simulink model "ODE_Hand_Model_v08_IPC_v03"  (Simulink 7.5)
settings: Solver=FixedStepDiscrete  StartTime=0.0  StopTime=inf  FixedStep=0.0315/(4*12)  RelTol=1e-3
values from neighbouring files (symbols this model uses):
  f_step = 0.7    [Set_Parameters.m]
  force_step = 20    [Set_Parameters.m]
  K_Conn = eye(4)*k_conn    [Set_Parameters.m]
  K_D = 30    [Set_Parameters.m]
  K_Or = eye(3)*k_Or    [Set_Parameters.m]
  K_Ot = eye(3)*k_Ot    [Set_Parameters.m]
  K_P = 350    [Set_Parameters.m]
  ksi = 0.9    [Set_Parameters.m]
  Kx = diag([diag(K_Ot)' diag(K_Or)' diag(K_Conn)'])    [Set_Parameters.m]
  l_des = [l1_des; l2_des; l3_des; l4_des]    [Set_Parameters.m]
  Mo = diag([sphere_mass*ones(1,3) (2/5)*sphere_mass*sphere_radius^2*ones(1,3)])    [Set_Parameters.m]
  qd_initial_touch = [0 0.3655   -0.5897   -0.5897     0       -0.3333   +0.5942   +0.5942         0       -0.298   --0.5226   --0.5226           0       -0.3333   +0.5942   +0.5942]    [Set_Parameters.m]
  R_O_Desired = R_O(x_i_v02(qd_initial_touch))    [Set_Parameters.m]
  t_f_start = 2.5    [Set_Parameters.m]
  torque_step = 60    [Set_Parameters.m]
  x_O_desired = (1/4)*sum(x_i_v02(qd_initial_touch))    [Set_Parameters.m]
undefined symbols (not defined in the file or in its folder): sigbuilder_block
libraries: dspmtrx3 x33, simulink x2, dspinverses x1
(part 6 of 6)

== matlab function Control/IPC/J/J_Or1/Embedded MATLAB Function2 ==
  data: xi input double size=[4 3]; J_r3 output double
%#eml
function J_r3 = partial_r3_to_x(xi)


x1 = xi(1,:)';
x2 = xi(2,:)';
x3 = xi(3,:)';
x4 = xi(4,:)';

r1=(( x1-x3 )/norm( x1-x3 ) + ...
    ( x2-x4 )/norm( x2-x4 ));


r1_unit=(r1/norm(r1));

r3 = skew( x1-x3 ) * ( x2-x4 );
r3_unit=r3/norm(r3);

r2_unit = skew(r3_unit)*r1_unit;

% RO=[r1_unit r2_unit r3_unit];


% partial_r3__term1 = (((norm(r3)^2)*eye(3)-(r3)*(r3)') / (norm((r3))^3));
partial_r3__term1 = (-skew(r3)^2)/(norm(r3)^3);

partial_r3__term2_x1x3 = skew(x2-x4)';
partial_r3__term2_x2x4 =  skew(x1-x3); 

partial_r3__term3_x1x2 =  eye(3);
partial_r3__term3_x3x4 = -eye(3);

J_r3_x1 = partial_r3__term1*partial_r3__term2_x1x3*partial_r3__term3_x1x2;

J_r3_x2 = partial_r3__term1*partial_r3__term2_x2x4*partial_r3__term3_x1x2;
       
J_r3_x3 = partial_r3__term1*partial_r3__term2_x1x3*partial_r3__term3_x3x4;
                    
J_r3_x4 = partial_r3__term1*partial_r3__term2_x2x4*partial_r3__term3_x3x4;


J_r3 = [J_r3_x1,J_r3_x2,J_r3_x3,J_r3_x4];

== matlab function Control/IPC/J/J_Or1/Embedded MATLAB Function3 ==
  data: xi input double size=[4 3]; J_r1 output double
%#eml
function J_r1 = partial_r1_to_x(xi)


x1 = xi(1,:)';
x2 = xi(2,:)';
x3 = xi(3,:)';
x4 = xi(4,:)';

r1=(( x1-x3 )/norm( x1-x3 ) + ( x2-x4 )/norm( x2-x4 ));

% r1=(( x1-x3 )/norm( x1-x3 ) + ( x2-x4 ))


r1_unit=(r1/norm(r1));

r3= skew( x1-x3 ) * ( x2-x4 );
r3_unit=r3/norm(r3);

r2_unit = skew(r3_unit)*r1_unit;

% RO=[r1_unit r2_unit r3_unit];


% partial_r1__term1 = (((norm(r1)^2)*eye(3)-(r1)*(r1)') / (norm((r1))^3));
partial_r1__term1 = (-skew(r1)^2)/(norm(r1)^3);

partial_r1__term2_x1x3 = (((norm((x1-x3))^2)*eye(3)-(x1-x3)*(x1-x3)') / (norm((x1-x3))^3));
partial_r1__term2_x2x4 = (((norm((x2-x4))^2)*eye(3)-(x2-x4)*(x2-x4)') / (norm((x2-x4))^3));


partial_r1__term3_x1x2 = eye(3);
partial_r1__term3_x3x4 = -eye(3);



J_r1_x1 = partial_r1__term1*partial_r1__term2_x1x3*partial_r1__term3_x1x2;

J_r2 = skew(r3_unit)*J_r1_x1';

J_r1_x2 = partial_r1__term1*partial_r1__term2_x2x4*partial_r1__term3_x1x2;
       
J_r1_x3 = partial_r1__term1*partial_r1__term2_x1x3*partial_r1__term3_x3x4;
       
J_r1_x4 = partial_r1__term1*partial_r1__term2_x2x4*partial_r1__term3_x3x4;


% J_r1_x1 = [partial_r1__term1.*partial_r1__term2_x1x3.*partial_r1__term3_x1x2(:,1), ...
%            partial_r1__term1.*partial_r1__term2_x1x3.*partial_r1__term3_x1x2(:,2), ...
%            partial_r1__term1.*partial_r1__term2_x1x3.*partial_r1__term3_x1x2(:,3)];
% 
% J_r1_x2 = [partial_r1__term1.*partial_r1__term2_x2x4.*partial_r1__term3_x1x2(:,1), ...
%            partial_r1__term1.*partial_r1__term2_x2x4.*partial_r1__term3_x1x2(:,2), ...
%            partial_r1__term1.*partial_r1__term2_x2x4.*partial_r1__term3_x1x2(:,3)];
%        
% J_r1_x3 = [partial_r1__term1.*partial_r1__term2_x1x3.*partial_r1__term3_x3x4(:,1), ...
%            partial_r1__term1.*partial_r1__term2_x1x3.*partial_r1__term3_x3x4(:,2), ...
%            partial_r1__term1.*partial_r1__term2_x1x3.*partial_r1__term3_x3x4(:,3)];
%        
% J_r1_x4 = [partial_r1__term1.*partial_r1__term2_x2x4.*partial_r1__term3_x3x4(:,1), ...
%            partial_r1__term1.*partial_r1__term2_x2x4.*partial_r1__term3_x3x4(:,2), ...
%            partial_r1__term1.*partial_r1__term2_x2x4.*partial_r1__term3_x3x4(:,3)];

J_r1 = [J_r1_x1,J_r1_x2,J_r1_x3,J_r1_x4];

== matlab function Control/IPC/Object Level Damping(theta)/Embedded MATLAB Function ==
  data: q input double; M output double
%#eml
function M=Inertia_Dynamic_Terms(q)

M1=zeros(16);

L1 = 0.10;
L2 = 1.10;
L3 = 0.60;
L4 = 0.55;

capsule1Inertia = 0.1675;
capsule2Inertia = 0.0837;
capsule3Inertia = 0.0834;

caspule1mass = 2.00;
caspule2mass = 1.00;
caspule3mass = 1.00;

for i=1:4:16,
q1 = q(i);
q2 = q(i+1);
q3 = q(i+2);
q4 = q(i+3);
    
    
M1(i:i+3,i:i+3)=[capsule1Inertia .* cos(q2) .^ 2 + capsule2Inertia .* cos(q2 + q3) ...
   .^ 2 + capsule3Inertia .* cos(q2 + q3 + q4) .^ 2 + caspule1mass  ...
  .* ((1 / 4) .* L2 .^ 2 .* cos(q1) .^ 2 .* cos(q2) .^ 2 + (1 / 4)  ...
  .* L2 .^ 2 .* cos(q2) .^ 2 .* sin(q1) .^ 2) + caspule2mass .* ((( ...
  -1 / 2) .* L3 .* cos(q1) .* cos(q2 + q3) + cos(q1) .* (L2 .* cos( ...
  q2) + L3 .* cos(q2 + q3))) .^ 2 + ((1 / 2) .* L3 .* cos(q2 + q3)  ...
  .* sin(q1) + (-1) .* (L2 .* cos(q2) + L3 .* cos(q2 + q3)) .* sin( ...
  q1)) .^ 2) + caspule3mass .* (((-1 / 2) .* L4 .* cos(q1) .* cos( ...
  q2 + q3 + q4) + cos(q1) .* (L2 .* cos(q2) + L3 .* cos(q2 + q3) +  ...
  L4 .* cos(q2 + q3 + q4))) .^ 2 + ((1 / 2) .* L4 .* cos(q2 + q3 +  ...
  q4) .* sin(q1) + (-1) .* (L2 .* cos(q2) + L3 .* cos(q2 + q3) + L4  ...
  .* cos(q2 + q3 + q4)) .* sin(q1)) .^ 2) + capsule1Inertia .* sin( ...
  q2) .^ 2 + capsule2Inertia .* sin(q2 + q3) .^ 2 + capsule3Inertia  ...
  .* sin(q2 + q3 + q4) .^ 2,caspule2mass .* ((-1) .* ((-1 / 2) .*  ...
  L3 .* cos(q1) .* cos(q2 + q3) + cos(q1) .* (L2 .* cos(q2) + L3 .*  ...
  cos(q2 + q3))) .* sin(q1) .* (L2 .* sin(q2) + (1 / 2) .* L3 .*  ...
  sin(q2 + q3)) + (-1) .* cos(q1) .* ((1 / 2) .* L3 .* cos(q2 + q3)  ...
  .* sin(q1) + (-1) .* (L2 .* cos(q2) + L3 .* cos(q2 + q3)) .* sin( ...
  q1)) .* (L2 .* sin(q2) + (1 / 2) .* L3 .* sin(q2 + q3))) +  ...
  caspule3mass .* ((-1) .* ((-1 / 2) .* L4 .* cos(q1) .* cos(q2 +  ...
  q3 + q4) + cos(q1) .* (L2 .* cos(q2) + L3 .* cos(q2 + q3) + L4 .*  ...
  cos(q2 + q3 + q4))) .* sin(q1) .* (L2 .* sin(q2) + L3 .* sin(q2 +  ...
  q3) + (1 / 2) .* L4 .* sin(q2 + q3 + q4)) + (-1) .* cos(q1) .* (( ...
  1 / 2) .* L4 .* cos(q2 + q3 + q4) .* sin(q1) + (-1) .* (L2 .* cos( ...
  q2) + L3 .* cos(q2 + q3) + L4 .* cos(q2 + q3 + q4)) .* sin(q1)) .* ...
   (L2 .* sin(q2) + L3 .* sin(q2 + q3) + (1 / 2) .* L4 .* sin(q2 +  ...
  q3 + q4))),caspule2mass .* ((-1 / 2) .* L3 .* ((-1 / 2) .* L3 .*  ...
  cos(q1) .* cos(q2 + q3) + cos(q1) .* (L2 .* cos(q2) + L3 .* cos( ...
  q2 + q3))) .* sin(q1) .* sin(q2 + q3) + (-1 / 2) .* L3 .* cos(q1)  ...
  .* ((1 / 2) .* L3 .* cos(q2 + q3) .* sin(q1) + (-1) .* (L2 .* cos( ...
  q2) + L3 .* cos(q2 + q3)) .* sin(q1)) .* sin(q2 + q3)) +  ...
  caspule3mass .* ((-1) .* ((-1 / 2) .* L4 .* cos(q1) .* cos(q2 +  ...
  q3 + q4) + cos(q1) .* (L2 .* cos(q2) + L3 .* cos(q2 + q3) + L4 .*  ...
  cos(q2 + q3 + q4))) .* sin(q1) .* (L3 .* sin(q2 + q3) + (1 / 2) .* ...
   L4 .* sin(q2 + q3 + q4)) + (-1) .* cos(q1) .* ((1 / 2) .* L4 .*  ...
  cos(q2 + q3 + q4) .* sin(q1) + (-1) .* (L2 .* cos(q2) + L3 .* cos( ...
  q2 + q3) + L4 .* cos(q2 + q3 + q4)) .* sin(q1)) .* (L3 .* sin(q2 + ...
   q3) + (1 / 2) .* L4 .* sin(q2 + q3 + q4))),caspule3mass .* ((-1  ...
  / 2) .* L4 .* ((-1 / 2) .* L4 .* cos(q1) .* cos(q2 + q3 + q4) +  ...
  cos(q1) .* (L2 .* cos(q2) + L3 .* cos(q2 + q3) + L4 .* cos(q2 +  ...
  q3 + q4))) .* sin(q1) .* sin(q2 + q3 + q4) + (-1 / 2) .* L4 .*  ...
  cos(q1) .* ((1 / 2) .* L4 .* cos(q2 + q3 + q4) .* sin(q1) + (-1)  ...
  .* (L2 .* cos(q2) + L3 .* cos(q2 + q3) + L4 .* cos(q2 + q3 + q4))  ...
  .* sin(q1)) .* sin(q2 + q3 + q4));caspule2mass .* ((-1) .* ((-1 /  ...
  2) .* L3 .* cos(q1) .* cos(q2 + q3) + cos(q1) .* (L2 .* cos(q2) +  ...
  L3 .* cos(q2 + q3))) .* sin(q1) .* (L2 .* sin(q2) + (1 / 2) .* L3  ...
  .* sin(q2 + q3)) + (-1) .* cos(q1) .* ((1 / 2) .* L3 .* cos(q2 +  ...
  q3) .* sin(q1) + (-1) .* (L2 .* cos(q2) + L3 .* cos(q2 + q3)) .*  ...
  sin(q1)) .* (L2 .* sin(q2) + (1 / 2) .* L3 .* sin(q2 + q3))) +  ...
  caspule3mass .* ((-1) .* ((-1 / 2) .* L4 .* cos(q1) .* cos(q2 +  ...
  q3 + q4) + cos(q1) .* (L2 .* cos(q2) + L3 .* cos(q2 + q3) + L4 .*  ...
  cos(q2 + q3 + q4))) .* sin(q1) .* (L2 .* sin(q2) + L3 .* sin(q2 +  ...
  q3) + (1 / 2) .* L4 .* sin(q2 + q3 + q4)) + (-1) .* cos(q1) .* (( ...
  1 / 2) .* L4 .* cos(q2 + q3 + q4) .* sin(q1) + (-1) .* (L2 .* cos( ...
  q2) + L3 .* cos(q2 + q3) + L4 .* cos(q2 + q3 + q4)) .* sin(q1)) .* ...
   (L2 .* sin(q2) + L3 .* sin(q2 + q3) + (1 / 2) .* L4 .* sin(q2 +  ...
  q3 + q4))),capsule1Inertia .* cos(q1) .^ 2 .* (cos(q1) .^ 2 + sin( ...
  q1) .^ 2) + capsule2Inertia .* cos(q1) .^ 2 .* (cos(q1) .^ 2 +  ...
  sin(q1) .^ 2) + capsule3Inertia .* cos(q1) .^ 2 .* (cos(q1) .^ 2 + ...
   sin(q1) .^ 2) + capsule1Inertia .* sin(q1) .^ 2 .* (cos(q1) .^ 2  ...
  + sin(q1) .^ 2) + capsule2Inertia .* sin(q1) .^ 2 .* (cos(q1) .^  ...
  2 + sin(q1) .^ 2) + capsule3Inertia .* sin(q1) .^ 2 .* (cos(q1)  ...
  .^ 2 + sin(q1) .^ 2) + caspule1mass .* (((1 / 2) .* L2 .* cos(q1)  ...
  .^ 2 .* cos(q2) + (1 / 2) .* L2 .* cos(q2) .* sin(q1) .^ 2) .^ 2 + ...
   (1 / 4) .* L2 .^ 2 .* cos(q1) .^ 2 .* sin(q2) .^ 2 + (1 / 4) .*  ...
  L2 .^ 2 .* sin(q1) .^ 2 .* sin(q2) .^ 2) + caspule2mass .* ((cos( ...
  q1) .* ((-1 / 2) .* L3 .* cos(q1) .* cos(q2 + q3) + cos(q1) .* ( ...
  L2 .* cos(q2) + L3 .* cos(q2 + q3))) + sin(q1) .* ((-1 / 2) .* L3  ...
  .* cos(q2 + q3) .* sin(q1) + (L2 .* cos(q2) + L3 .* cos(q2 + q3))  ...
  .* sin(q1))) .^ 2 + cos(q1) .^ 2 .* (L2 .* sin(q2) + (1 / 2) .*  ...
  L3 .* sin(q2 + q3)) .^ 2 + sin(q1) .^ 2 .* (L2 .* sin(q2) + (1 /  ...
  2) .* L3 .* sin(q2 + q3)) .^ 2) + caspule3mass .* ((cos(q1) .* (( ...
  -1 / 2) .* L4 .* cos(q1) .* cos(q2 + q3 + q4) + cos(q1) .* (L2 .*  ...
  cos(q2) + L3 .* cos(q2 + q3) + L4 .* cos(q2 + q3 + q4))) + sin(q1) ...
   .* ((-1 / 2) .* L4 .* cos(q2 + q3 + q4) .* sin(q1) + (L2 .* cos( ...
  q2) + L3 .* cos(q2 + q3) + L4 .* cos(q2 + q3 + q4)) .* sin(q1)))  ...
  .^ 2 + cos(q1) .^ 2 .* (L2 .* sin(q2) + L3 .* sin(q2 + q3) + (1 /  ...
  2) .* L4 .* sin(q2 + q3 + q4)) .^ 2 + sin(q1) .^ 2 .* (L2 .* sin( ...
  q2) + L3 .* sin(q2 + q3) + (1 / 2) .* L4 .* sin(q2 + q3 + q4)) .^  ...
  2),capsule2Inertia .* cos(q1) .^ 2 .* (cos(q1) .^ 2 + sin(q1) .^  ...
  2) + capsule3Inertia .* cos(q1) .^ 2 .* (cos(q1) .^ 2 + sin(q1)  ...
  .^ 2) + capsule2Inertia .* sin(q1) .^ 2 .* (cos(q1) .^ 2 + sin(q1) ...
   .^ 2) + capsule3Inertia .* sin(q1) .^ 2 .* (cos(q1) .^ 2 + sin( ...
  q1) .^ 2) + caspule2mass .* ((cos(q1) .* ((-1 / 2) .* L3 .* cos( ...
  q1) .* cos(q2 + q3) + cos(q1) .* (L2 .* cos(q2) + L3 .* cos(q2 +  ...
  q3))) + sin(q1) .* ((-1 / 2) .* L3 .* cos(q2 + q3) .* sin(q1) + ( ...
  L2 .* cos(q2) + L3 .* cos(q2 + q3)) .* sin(q1))) .* (cos(q1) .* (( ...
  -1) .* L2 .* cos(q1) .* cos(q2) + (-1 / 2) .* L3 .* cos(q1) .*  ...
  cos(q2 + q3) + cos(q1) .* (L2 .* cos(q2) + L3 .* cos(q2 + q3))) +  ...
  sin(q1) .* ((-1) .* L2 .* cos(q2) .* sin(q1) + (-1 / 2) .* L3 .*  ...
  cos(q2 + q3) .* sin(q1) + (L2 .* cos(q2) + L3 .* cos(q2 + q3)) .*  ...
  sin(q1))) + (1 / 2) .* L3 .* cos(q1) .^ 2 .* sin(q2 + q3) .* (L2  ...
  .* sin(q2) + (1 / 2) .* L3 .* sin(q2 + q3)) + (1 / 2) .* L3 .*  ...
  sin(q1) .^ 2 .* sin(q2 + q3) .* (L2 .* sin(q2) + (1 / 2) .* L3 .*  ...
  sin(q2 + q3))) + caspule3mass .* ((cos(q1) .* ((-1 / 2) .* L4 .*  ...
  cos(q1) .* cos(q2 + q3 + q4) + cos(q1) .* (L2 .* cos(q2) + L3 .*  ...
  cos(q2 + q3) + L4 .* cos(q2 + q3 + q4))) + sin(q1) .* ((-1 / 2) .* ...
   L4 .* cos(q2 + q3 + q4) .* sin(q1) + (L2 .* cos(q2) + L3 .* cos( ...
  q2 + q3) + L4 .* cos(q2 + q3 + q4)) .* sin(q1))) .* (cos(q1) .* (( ...
  -1) .* L2 .* cos(q1) .* cos(q2) + (-1 / 2) .* L4 .* cos(q1) .*  ...
  cos(q2 + q3 + q4) + cos(q1) .* (L2 .* cos(q2) + L3 .* cos(q2 + q3) ...
   + L4 .* cos(q2 + q3 + q4))) + sin(q1) .* ((-1) .* L2 .* cos(q2)  ...
  .* sin(q1) + (-1 / 2) .* L4 .* cos(q2 + q3 + q4) .* sin(q1) + (L2  ...
  .* cos(q2) + L3 .* cos(q2 + q3) + L4 .* cos(q2 + q3 + q4)) .* sin( ...
  q1))) + cos(q1) .^ 2 .* (L3 .* sin(q2 + q3) + (1 / 2) .* L4 .*  ...
  sin(q2 + q3 + q4)) .* (L2 .* sin(q2) + L3 .* sin(q2 + q3) + (1 /  ...
  2) .* L4 .* sin(q2 + q3 + q4)) + sin(q1) .^ 2 .* (L3 .* sin(q2 +  ...
  q3) + (1 / 2) .* L4 .* sin(q2 + q3 + q4)) .* (L2 .* sin(q2) + L3  ...
  .* sin(q2 + q3) + (1 / 2) .* L4 .* sin(q2 + q3 + q4))), ...
  capsule3Inertia .* cos(q1) .^ 2 .* (cos(q1) .^ 2 + sin(q1) .^ 2) + ...
   capsule3Inertia .* sin(q1) .^ 2 .* (cos(q1) .^ 2 + sin(q1) .^ 2)  ...
  + caspule3mass .* ((cos(q1) .* ((-1 / 2) .* L4 .* cos(q1) .* cos( ...
  q2 + q3 + q4) + cos(q1) .* (L2 .* cos(q2) + L3 .* cos(q2 + q3) +  ...
  L4 .* cos(q2 + q3 + q4))) + sin(q1) .* ((-1 / 2) .* L4 .* cos(q2 + ...
   q3 + q4) .* sin(q1) + (L2 .* cos(q2) + L3 .* cos(q2 + q3) + L4 .* ...
   cos(q2 + q3 + q4)) .* sin(q1))) .* (cos(q1) .* ((-1) .* cos(q1)  ...
  .* (L2 .* cos(q2) + L3 .* cos(q2 + q3)) + (-1 / 2) .* L4 .* cos( ...
  q1) .* cos(q2 + q3 + q4) + cos(q1) .* (L2 .* cos(q2) + L3 .* cos( ...
  q2 + q3) + L4 .* cos(q2 + q3 + q4))) + sin(q1) .* ((-1) .* (L2 .*  ...
  cos(q2) + L3 .* cos(q2 + q3)) .* sin(q1) + (-1 / 2) .* L4 .* cos( ...
  q2 + q3 + q4) .* sin(q1) + (L2 .* cos(q2) + L3 .* cos(q2 + q3) +  ...
  L4 .* cos(q2 + q3 + q4)) .* sin(q1))) + (1 / 2) .* L4 .* cos(q1)  ...
  .^ 2 .* sin(q2 + q3 + q4) .* (L2 .* sin(q2) + L3 .* sin(q2 + q3) + ...
   (1 / 2) .* L4 .* sin(q2 + q3 + q4)) + (1 / 2) .* L4 .* sin(q1)  ...
  .^ 2 .* sin(q2 + q3 + q4) .* (L2 .* sin(q2) + L3 .* sin(q2 + q3) + ...
   (1 / 2) .* L4 .* sin(q2 + q3 + q4)));caspule2mass .* ((-1 / 2) .* ...
   L3 .* ((-1 / 2) .* L3 .* cos(q1) .* cos(q2 + q3) + cos(q1) .* ( ...
  L2 .* cos(q2) + L3 .* cos(q2 + q3))) .* sin(q1) .* sin(q2 + q3) +  ...
  (-1 / 2) .* L3 .* cos(q1) .* ((1 / 2) .* L3 .* cos(q2 + q3) .*  ...
  sin(q1) + (-1) .* (L2 .* cos(q2) + L3 .* cos(q2 + q3)) .* sin(q1)) ...
   .* sin(q2 + q3)) + caspule3mass .* ((-1) .* ((-1 / 2) .* L4 .*  ...
  cos(q1) .* cos(q2 + q3 + q4) + cos(q1) .* (L2 .* cos(q2) + L3 .*  ...
  cos(q2 + q3) + L4 .* cos(q2 + q3 + q4))) .* sin(q1) .* (L3 .* sin( ...
  q2 + q3) + (1 / 2) .* L4 .* sin(q2 + q3 + q4)) + (-1) .* cos(q1)  ...
  .* ((1 / 2) .* L4 .* cos(q2 + q3 + q4) .* sin(q1) + (-1) .* (L2 .* ...
   cos(q2) + L3 .* cos(q2 + q3) + L4 .* cos(q2 + q3 + q4)) .* sin( ...
  q1)) .* (L3 .* sin(q2 + q3) + (1 / 2) .* L4 .* sin(q2 + q3 + q4))) ...
  ,capsule2Inertia .* cos(q1) .^ 2 .* (cos(q1) .^ 2 + sin(q1) .^ 2)  ...
  + capsule3Inertia .* cos(q1) .^ 2 .* (cos(q1) .^ 2 + sin(q1) .^ 2) ...
   + capsule2Inertia .* sin(q1) .^ 2 .* (cos(q1) .^ 2 + sin(q1) .^  ...
  2) + capsule3Inertia .* sin(q1) .^ 2 .* (cos(q1) .^ 2 + sin(q1)  ...
  .^ 2) + caspule2mass .* ((cos(q1) .* ((-1 / 2) .* L3 .* cos(q1) .* ...
   cos(q2 + q3) + cos(q1) .* (L2 .* cos(q2) + L3 .* cos(q2 + q3))) + ...
   sin(q1) .* ((-1 / 2) .* L3 .* cos(q2 + q3) .* sin(q1) + (L2 .*  ...
  cos(q2) + L3 .* cos(q2 + q3)) .* sin(q1))) .* (cos(q1) .* ((-1) .* ...
   L2 .* cos(q1) .* cos(q2) + (-1 / 2) .* L3 .* cos(q1) .* cos(q2 +  ...
  q3) + cos(q1) .* (L2 .* cos(q2) + L3 .* cos(q2 + q3))) + sin(q1)  ...
  .* ((-1) .* L2 .* cos(q2) .* sin(q1) + (-1 / 2) .* L3 .* cos(q2 +  ...
  q3) .* sin(q1) + (L2 .* cos(q2) + L3 .* cos(q2 + q3)) .* sin(q1))) ...
   + (1 / 2) .* L3 .* cos(q1) .^ 2 .* sin(q2 + q3) .* (L2 .* sin(q2) ...
   + (1 / 2) .* L3 .* sin(q2 + q3)) + (1 / 2) .* L3 .* sin(q1) .^ 2  ...
  .* sin(q2 + q3) .* (L2 .* sin(q2) + (1 / 2) .* L3 .* sin(q2 + q3)) ...
  ) + caspule3mass .* ((cos(q1) .* ((-1 / 2) .* L4 .* cos(q1) .*  ...
  cos(q2 + q3 + q4) + cos(q1) .* (L2 .* cos(q2) + L3 .* cos(q2 + q3) ...
   + L4 .* cos(q2 + q3 + q4))) + sin(q1) .* ((-1 / 2) .* L4 .* cos( ...
  q2 + q3 + q4) .* sin(q1) + (L2 .* cos(q2) + L3 .* cos(q2 + q3) +  ...
  L4 .* cos(q2 + q3 + q4)) .* sin(q1))) .* (cos(q1) .* ((-1) .* L2  ...
  .* cos(q1) .* cos(q2) + (-1 / 2) .* L4 .* cos(q1) .* cos(q2 + q3 + ...
   q4) + cos(q1) .* (L2 .* cos(q2) + L3 .* cos(q2 + q3) + L4 .* cos( ...
  q2 + q3 + q4))) + sin(q1) .* ((-1) .* L2 .* cos(q2) .* sin(q1) + ( ...
  -1 / 2) .* L4 .* cos(q2 + q3 + q4) .* sin(q1) + (L2 .* cos(q2) +  ...
  L3 .* cos(q2 + q3) + L4 .* cos(q2 + q3 + q4)) .* sin(q1))) + cos( ...
  q1) .^ 2 .* (L3 .* sin(q2 + q3) + (1 / 2) .* L4 .* sin(q2 + q3 +  ...
  q4)) .* (L2 .* sin(q2) + L3 .* sin(q2 + q3) + (1 / 2) .* L4 .*  ...
  sin(q2 + q3 + q4)) + sin(q1) .^ 2 .* (L3 .* sin(q2 + q3) + (1 / 2) ...
   .* L4 .* sin(q2 + q3 + q4)) .* (L2 .* sin(q2) + L3 .* sin(q2 +  ...
  q3) + (1 / 2) .* L4 .* sin(q2 + q3 + q4))),capsule2Inertia .* cos( ...
  q1) .^ 2 .* (cos(q1) .^ 2 + sin(q1) .^ 2) + capsule3Inertia .*  ...
  cos(q1) .^ 2 .* (cos(q1) .^ 2 + sin(q1) .^ 2) + capsule2Inertia .* ...
   sin(q1) .^ 2 .* (cos(q1) .^ 2 + sin(q1) .^ 2) + capsule3Inertia  ...
  .* sin(q1) .^ 2 .* (cos(q1) .^ 2 + sin(q1) .^ 2) + caspule2mass .* ...
   ((cos(q1) .* ((-1) .* L2 .* cos(q1) .* cos(q2) + (-1 / 2) .* L3  ...
  .* cos(q1) .* cos(q2 + q3) + cos(q1) .* (L2 .* cos(q2) + L3 .*  ...
  cos(q2 + q3))) + sin(q1) .* ((-1) .* L2 .* cos(q2) .* sin(q1) + ( ...
  -1 / 2) .* L3 .* cos(q2 + q3) .* sin(q1) + (L2 .* cos(q2) + L3 .*  ...
  cos(q2 + q3)) .* sin(q1))) .^ 2 + (1 / 4) .* L3 .^ 2 .* cos(q1)  ...
  .^ 2 .* sin(q2 + q3) .^ 2 + (1 / 4) .* L3 .^ 2 .* sin(q1) .^ 2 .*  ...
  sin(q2 + q3) .^ 2) + caspule3mass .* ((cos(q1) .* ((-1) .* L2 .*  ...
  cos(q1) .* cos(q2) + (-1 / 2) .* L4 .* cos(q1) .* cos(q2 + q3 +  ...
  q4) + cos(q1) .* (L2 .* cos(q2) + L3 .* cos(q2 + q3) + L4 .* cos( ...
  q2 + q3 + q4))) + sin(q1) .* ((-1) .* L2 .* cos(q2) .* sin(q1) + ( ...
  -1 / 2) .* L4 .* cos(q2 + q3 + q4) .* sin(q1) + (L2 .* cos(q2) +  ...
  L3 .* cos(q2 + q3) + L4 .* cos(q2 + q3 + q4)) .* sin(q1))) .^ 2 +  ...
  cos(q1) .^ 2 .* (L3 .* sin(q2 + q3) + (1 / 2) .* L4 .* sin(q2 +  ...
  q3 + q4)) .^ 2 + sin(q1) .^ 2 .* (L3 .* sin(q2 + q3) + (1 / 2) .*  ...
  L4 .* sin(q2 + q3 + q4)) .^ 2),capsule3Inertia .* cos(q1) .^ 2 .*  ...
  (cos(q1) .^ 2 + sin(q1) .^ 2) + capsule3Inertia .* sin(q1) .^ 2 .* ...
   (cos(q1) .^ 2 + sin(q1) .^ 2) + caspule3mass .* ((cos(q1) .* (( ...
  -1) .* L2 .* cos(q1) .* cos(q2) + (-1 / 2) .* L4 .* cos(q1) .*  ...
  cos(q2 + q3 + q4) + cos(q1) .* (L2 .* cos(q2) + L3 .* cos(q2 + q3) ...
   + L4 .* cos(q2 + q3 + q4))) + sin(q1) .* ((-1) .* L2 .* cos(q2)  ...
  .* sin(q1) + (-1 / 2) .* L4 .* cos(q2 + q3 + q4) .* sin(q1) + (L2  ...
  .* cos(q2) + L3 .* cos(q2 + q3) + L4 .* cos(q2 + q3 + q4)) .* sin( ...
  q1))) .* (cos(q1) .* ((-1) .* cos(q1) .* (L2 .* cos(q2) + L3 .*  ...
  cos(q2 + q3)) + (-1 / 2) .* L4 .* cos(q1) .* cos(q2 + q3 + q4) +  ...
  cos(q1) .* (L2 .* cos(q2) + L3 .* cos(q2 + q3) + L4 .* cos(q2 +  ...
  q3 + q4))) + sin(q1) .* ((-1) .* (L2 .* cos(q2) + L3 .* cos(q2 +  ...
  q3)) .* sin(q1) + (-1 / 2) .* L4 .* cos(q2 + q3 + q4) .* sin(q1) + ...
   (L2 .* cos(q2) + L3 .* cos(q2 + q3) + L4 .* cos(q2 + q3 + q4)) .* ...
   sin(q1))) + (1 / 2) .* L4 .* cos(q1) .^ 2 .* sin(q2 + q3 + q4) .* ...
   (L3 .* sin(q2 + q3) + (1 / 2) .* L4 .* sin(q2 + q3 + q4)) + (1 /  ...
  2) .* L4 .* sin(q1) .^ 2 .* sin(q2 + q3 + q4) .* (L3 .* sin(q2 +  ...
  q3) + (1 / 2) .* L4 .* sin(q2 + q3 + q4)));caspule3mass .* ((-1 /  ...
  2) .* L4 .* ((-1 / 2) .* L4 .* cos(q1) .* cos(q2 + q3 + q4) + cos( ...
  q1) .* (L2 .* cos(q2) + L3 .* cos(q2 + q3) + L4 .* cos(q2 + q3 +  ...
  q4))) .* sin(q1) .* sin(q2 + q3 + q4) + (-1 / 2) .* L4 .* cos(q1)  ...
  .* ((1 / 2) .* L4 .* cos(q2 + q3 + q4) .* sin(q1) + (-1) .* (L2 .* ...
   cos(q2) + L3 .* cos(q2 + q3) + L4 .* cos(q2 + q3 + q4)) .* sin( ...
  q1)) .* sin(q2 + q3 + q4)),capsule3Inertia .* cos(q1) .^ 2 .* ( ...
  cos(q1) .^ 2 + sin(q1) .^ 2) + capsule3Inertia .* sin(q1) .^ 2 .*  ...
  (cos(q1) .^ 2 + sin(q1) .^ 2) + caspule3mass .* ((cos(q1) .* ((-1  ...
  / 2) .* L4 .* cos(q1) .* cos(q2 + q3 + q4) + cos(q1) .* (L2 .*  ...
  cos(q2) + L3 .* cos(q2 + q3) + L4 .* cos(q2 + q3 + q4))) + sin(q1) ...
   .* ((-1 / 2) .* L4 .* cos(q2 + q3 + q4) .* sin(q1) + (L2 .* cos( ...
  q2) + L3 .* cos(q2 + q3) + L4 .* cos(q2 + q3 + q4)) .* sin(q1)))  ...
  .* (cos(q1) .* ((-1) .* cos(q1) .* (L2 .* cos(q2) + L3 .* cos(q2 + ...
   q3)) + (-1 / 2) .* L4 .* cos(q1) .* cos(q2 + q3 + q4) + cos(q1)  ...
  .* (L2 .* cos(q2) + L3 .* cos(q2 + q3) + L4 .* cos(q2 + q3 + q4))) ...
   + sin(q1) .* ((-1) .* (L2 .* cos(q2) + L3 .* cos(q2 + q3)) .*  ...
  sin(q1) + (-1 / 2) .* L4 .* cos(q2 + q3 + q4) .* sin(q1) + (L2 .*  ...
  cos(q2) + L3 .* cos(q2 + q3) + L4 .* cos(q2 + q3 + q4)) .* sin(q1) ...
  )) + (1 / 2) .* L4 .* cos(q1) .^ 2 .* sin(q2 + q3 + q4) .* (L2 .*  ...
  sin(q2) + L3 .* sin(q2 + q3) + (1 / 2) .* L4 .* sin(q2 + q3 + q4)) ...
   + (1 / 2) .* L4 .* sin(q1) .^ 2 .* sin(q2 + q3 + q4) .* (L2 .*  ...
  sin(q2) + L3 .* sin(q2 + q3) + (1 / 2) .* L4 .* sin(q2 + q3 + q4)) ...
  ),capsule3Inertia .* cos(q1) .^ 2 .* (cos(q1) .^ 2 + sin(q1) .^ 2) ...
   + capsule3Inertia .* sin(q1) .^ 2 .* (cos(q1) .^ 2 + sin(q1) .^  ...
  2) + caspule3mass .* ((cos(q1) .* ((-1) .* L2 .* cos(q1) .* cos( ...
  q2) + (-1 / 2) .* L4 .* cos(q1) .* cos(q2 + q3 + q4) + cos(q1) .*  ...
  (L2 .* cos(q2) + L3 .* cos(q2 + q3) + L4 .* cos(q2 + q3 + q4))) +  ...
  sin(q1) .* ((-1) .* L2 .* cos(q2) .* sin(q1) + (-1 / 2) .* L4 .*  ...
  cos(q2 + q3 + q4) .* sin(q1) + (L2 .* cos(q2) + L3 .* cos(q2 + q3) ...
   + L4 .* cos(q2 + q3 + q4)) .* sin(q1))) .* (cos(q1) .* ((-1) .*  ...
  cos(q1) .* (L2 .* cos(q2) + L3 .* cos(q2 + q3)) + (-1 / 2) .* L4  ...
  .* cos(q1) .* cos(q2 + q3 + q4) + cos(q1) .* (L2 .* cos(q2) + L3  ...
  .* cos(q2 + q3) + L4 .* cos(q2 + q3 + q4))) + sin(q1) .* ((-1) .*  ...
  (L2 .* cos(q2) + L3 .* cos(q2 + q3)) .* sin(q1) + (-1 / 2) .* L4  ...
  .* cos(q2 + q3 + q4) .* sin(q1) + (L2 .* cos(q2) + L3 .* cos(q2 +  ...
  q3) + L4 .* cos(q2 + q3 + q4)) .* sin(q1))) + (1 / 2) .* L4 .*  ...
  cos(q1) .^ 2 .* sin(q2 + q3 + q4) .* (L3 .* sin(q2 + q3) + (1 / 2) ...
   .* L4 .* sin(q2 + q3 + q4)) + (1 / 2) .* L4 .* sin(q1) .^ 2 .*  ...
  sin(q2 + q3 + q4) .* (L3 .* sin(q2 + q3) + (1 / 2) .* L4 .* sin( ...
  q2 + q3 + q4))),capsule3Inertia .* cos(q1) .^ 2 .* (cos(q1) .^ 2 + ...
   sin(q1) .^ 2) + capsule3Inertia .* sin(q1) .^ 2 .* (cos(q1) .^ 2  ...
  + sin(q1) .^ 2) + caspule3mass .* ((cos(q1) .* ((-1) .* cos(q1) .* ...
   (L2 .* cos(q2) + L3 .* cos(q2 + q3)) + (-1 / 2) .* L4 .* cos(q1)  ...
  .* cos(q2 + q3 + q4) + cos(q1) .* (L2 .* cos(q2) + L3 .* cos(q2 +  ...
  q3) + L4 .* cos(q2 + q3 + q4))) + sin(q1) .* ((-1) .* (L2 .* cos( ...
  q2) + L3 .* cos(q2 + q3)) .* sin(q1) + (-1 / 2) .* L4 .* cos(q2 +  ...
  q3 + q4) .* sin(q1) + (L2 .* cos(q2) + L3 .* cos(q2 + q3) + L4 .*  ...
  cos(q2 + q3 + q4)) .* sin(q1))) .^ 2 + (1 / 4) .* L4 .^ 2 .* cos( ...
  q1) .^ 2 .* sin(q2 + q3 + q4) .^ 2 + (1 / 4) .* L4 .^ 2 .* sin(q1) ...
   .^ 2 .* sin(q2 + q3 + q4) .^ 2)];
end
M=M1;

== matlab function Control/IPC/Object Level Damping(theta)/Embedded MATLAB Function1 ==
  data: u input double; y output double
function y = fcn(u)
%#eml

y = inv(u);

== matlab function Control/IPC/J/J_Ot1/Embedded MATLAB Function ==
  data: u input double; y output double
function y = fcn(u)
%#eml

y = (u(1,:)+u(2,:)+u(3,:)+u(4,:))/4;

== matlab function Control/IPC/J/J_Ot1/Embedded MATLAB Function1 ==
  data: v_in input double size=[3 1]; S output double
%#eml
function S = skew(v_in)

v=v_in';
    S = [  0   -v(1,3)  v(1,2);
          v(1,3)  0    -v(1,1);
          -v(1,2) v(1,1)   0];

== matlab function Control/IPC/J/J_Or1/Embedded MATLAB Function ==
  data: u input double size=[3 3]; y output double
function y = fcn(u)
%#eml

y = u(:,1)';

== matlab function Control/IPC/J/J_Or1/Embedded MATLAB Function4 ==
  data: u input double size=[3 3]; y output double
function y = fcn(u)
%#eml

y = u(:,2)';

== matlab function Control/IPC/J/J_Or1/Embedded MATLAB Function5 ==
  data: u input double size=[3 3]; y output double
function y = fcn(u)
%#eml

y = u(:,3)';

== matlab function Control/IPC/J/Jconn/Embedded MATLAB Function ==
  data: xi input double size=[4 3]; Jc output double
%#eml
function Jc=partial_x(xi)

dx =zeros(4,3);
norm_dx=zeros(1,4);


b=(1-(1/4));
a=-1/4;
% a=0;


x1 = xi(1,:);
x2 = xi(2,:);
x3 = xi(3,:);
x4 = xi(4,:);


xO = (1/4)*(x1+x2+x3+x4);
% xO = [0.2000         0    2.09];

% 
dx(1,:)=((x1-xO));
dx(2,:)=((x2-xO));
dx(3,:)=((x3-xO));
dx(4,:)=((x4-xO));

norm_dx(1) = norm(dx(1,:));
norm_dx(2) = norm(dx(2,:));
norm_dx(3) = norm(dx(3,:));
norm_dx(4) = norm(dx(4,:));

partial_delta_x1 = [b*eye(3); a*eye(3); a*eye(3); a*eye(3)];

partial_delta_x2 = [a*eye(3); b*eye(3); a*eye(3); a*eye(3)];

partial_delta_x3 = [a*eye(3); a*eye(3); b*eye(3); a*eye(3)];

partial_delta_x4 = [a*eye(3); a*eye(3); a*eye(3); b*eye(3)];


% size(partial_delta_x1)
% size(dx(1,:))
% size(norm_dx(1))

Jc=[partial_delta_x1*(dx(1,:)'/norm_dx(1)), partial_delta_x2*(dx(2,:)'/norm_dx(2)), ...
    partial_delta_x3*(dx(3,:)'/norm_dx(3)), partial_delta_x4*(dx(4,:)'/norm_dx(4))];

== matlab function Initialization & Object Level Path Planning/Embedded MATLAB Function1 ==
  data: xi input double size=[4 3]; RO output double
%#eml
function RO=R_O(xi)



x1 = xi(1,:);
x2 = xi(2,:);
x3 = xi(3,:);
x4 = xi(4,:);

% r1=( xi(1,:)-xi(3,:) )/norm( xi(1,:)-xi(3,:) ) + ...
%     ( xi(2,:)-xi(4,:) )/norm( xi(2,:)-xi(4,:) );

r1=( x1-x3 )/norm( x1-x3 ) + ...
    ( x2-x4 )/norm( x2-x4 );


r1_unit=r1/norm(r1);

% r3= cross( (x1-x3),( x2-x4 ))';

r3= skew( x1-x3 ) * ( x2-x4 )';
r3_unit=r3/norm(r3);

r2_unit = skew(r3_unit)*r1_unit';

l=[r1_unit' r2_unit r3_unit];
RO=l;

== matlab function Initialization & Object Level Path Planning/Embedded MATLAB Function2 ==
  data: q input double; x output double
%#eml
function x=x_i_v02(q)

x_=zeros(4,3);

rot_base=[0.0000         0   -1.0000;
         0    1.0000         0;
    1.0000         0    0.0000];

L1 = 0.10;
L2 = 1.10;
L3 = 0.60;
L4 = 0.55;

fingers_positions = [-0.70,   0,  L1;...
                      0.60,  0.40,  L1;...
                      0.70,   0,  L1;...
                      0.60,  -0.40, L1];

c=1;
                  
for i=1:4:16,

q1 = q(i);
q2 = q(i+1);
q3 = q(i+2);
q4 = q(i+3);

x_(c,1)=cos(q1) .* (L2 .* cos(q2) + L3 .* cos(q2 + q3) + L4 .*  cos(q2 + q3 + q4));
x_(c,2)=(L2 .* cos(q2) + L3 .* cos(q2 + q3) + L4 .* cos(q2 + q3 + q4)) .* sin(q1);
x_(c,3)= L2 .* sin(q2) + L3 .* sin(q2 + q3) + L4 .* sin(q2 + q3 + q4);

x_(c,:)=rot_base*x_(c,:)'+fingers_positions(c,:)';
c=c+1;
end

x=x_;

== matlab function Control/IPC/Finger Redundancy Controller/Embedded MATLAB Function ==
  data: q_in input double size=[1,16]; tau_N output double; dq_in input double size=[1,16]
%#eml
function tau_N = redundancy_controller(q_in,dq_in)

q=q_in;
dq=dq_in';

J=zeros(24,16);

L2 = 1.10;
L3 = 0.60;
L4 = 0.55;

rot_base1=[0.0000         0   -1.0000;
         0    1.0000         0;
    1.0000         0    0.0000];

rot_base=[rot_base1,zeros(3);zeros(3), rot_base1];

c=1;
for i=1:4:16
q1 = q(i);
q2 = q(i+1);
q3 = q(i+2);
q4 = q(i+3);


J(c:c+5,i:i+3)=rot_base*[(-1) .* (L2 .* cos(q2) + L3 .* cos(q2 + q3) + L4 .* cos(q2 + q3 + ...
   q4)) .* sin(q1),(-1) .* cos(q1) .* (L2 .* sin(q2) + L3 .* sin(q2  ...
  + q3) + L4 .* sin(q2 + q3 + q4)),(-1) .* cos(q1) .* (L3 .* sin(q2  ...
  + q3) + L4 .* sin(q2 + q3 + q4)),(-1) .* L4 .* cos(q1) .* sin(q2 + ...
   q3 + q4);cos(q1) .* (L2 .* cos(q2) + L3 .* cos(q2 + q3) + L4 .*  ...
  cos(q2 + q3 + q4)),(-1) .* sin(q1) .* (L2 .* sin(q2) + L3 .* sin( ...
  q2 + q3) + L4 .* sin(q2 + q3 + q4)),(-1) .* sin(q1) .* (L3 .* sin( ...
  q2 + q3) + L4 .* sin(q2 + q3 + q4)),(-1) .* L4 .* sin(q1) .* sin( ...
  q2 + q3 + q4);0,cos(q1) .^ 2 .* (L2 .* cos(q2) + L3 .* cos(q2 +  ...
  q3) + L4 .* cos(q2 + q3 + q4)) + (L2 .* cos(q2) + L3 .* cos(q2 +  ...
  q3) + L4 .* cos(q2 + q3 + q4)) .* sin(q1) .^ 2,cos(q1) .* ((-1) .* ...
   L2 .* cos(q1) .* cos(q2) + cos(q1) .* (L2 .* cos(q2) + L3 .* cos( ...
  q2 + q3) + L4 .* cos(q2 + q3 + q4))) + sin(q1) .* ((-1) .* L2 .*  ...
  cos(q2) .* sin(q1) + (L2 .* cos(q2) + L3 .* cos(q2 + q3) + L4 .*  ...
  cos(q2 + q3 + q4)) .* sin(q1)),cos(q1) .* ((-1) .* cos(q1) .* (L2  ...
  .* cos(q2) + L3 .* cos(q2 + q3)) + cos(q1) .* (L2 .* cos(q2) + L3  ...
  .* cos(q2 + q3) + L4 .* cos(q2 + q3 + q4))) + sin(q1) .* ((-1) .*  ...
  (L2 .* cos(q2) + L3 .* cos(q2 + q3)) .* sin(q1) + (L2 .* cos(q2) + ...
   L3 .* cos(q2 + q3) + L4 .* cos(q2 + q3 + q4)) .* sin(q1));0,sin( ...
  q1),sin(q1),sin(q1);0,(-1) .* cos(q1),(-1) .* cos(q1),(-1) .* cos( ...
  q1);1,0,0,0];

c=c+6;
end
JH=J;


% size(JH)
K_P=50;
K_D=0.9;
%  K=0;
a=1;
tau = zeros(1,16);

for i=1:4:16
    tau(i:i+3) = (K_P*(q(i+2)-a*q(i+3)))*[0 0 1 -1]+K_D*(dq(i:i+3)');
end

tau_N=(eye(16)-JH'*JH)*tau';

== matlab function Control/IPC/Object Level Stiffnes /VO,r(theta)/Embedded MATLAB Function2 ==
  data: e input double; J output double
%#eml
function J=Jwe(e)





q0 = e(1); 
q1 = e(2);
q2 = e(3);
q3 = e(4);



% R_O_Desired=[-0.7071    0.7071         0; ...
%     0.7071    0.7071         0; ...
%          0         0   -1.0000];



J = -4*(1/2)*[q0 -q3  q2;...
             q3  q0 -q1;...
            -q2  q1  q0];

== matlab function Control/IPC/Object Level Stiffnes /VConn(theta)/Embedded MATLAB Function ==
  data: xi input double size=[4 3]; Deltax output double
%#eml
function Deltax=Delta_x(xi)

dx = zeros(1,4);

x1 = xi(1,:);
x2 = xi(2,:);
x3 = xi(3,:);
x4 = xi(4,:);


xO = (1/4)*(x1+x2+x3+x4);
% xO =[0.2000         0    2.0900];


% 
dx(1)=norm((x1-xO));
dx(2)=norm((x2-xO));
dx(3)=norm((x3-xO));
dx(4)=norm((x4-xO));

Deltax=dx';

== matlab function Control/IPC/Object Level Stiffnes /VO,t(theta)/Embedded MATLAB Function ==
  data: u input double size=[4 3]; y output double
function y = fcn(u)
%#eml

y = ((u(1,:)+u(2,:)+u(3,:)+u(4,:))/4)';

== matlab function Initialization & Object Level Path Planning/q Desired/Embedded MATLAB Function ==
  data: key input double size=1; x_f output double size=[1 3]; r_f output double size=[1 3]
function [x_f,r_f]=q_d(key)

% torque_signal_out=zeros(1,16);
x=zeros(1,3);
r=zeros(1,3);

q_incr=0.01;
% q_incr = pi/8;
current_key=key;

switch current_key
   case 30
      x(1)=q_incr;
   case 31
      x(1)=-q_incr;
   case 28
      x(2)=q_incr;
   case 29
      x(2)=-q_incr;   
   case 56
      x(3)=q_incr;
   case 50
      x(3)=-q_incr;
   case uint8('w')
      r(1)=q_incr;
   case uint8('x')
      r(1)=-q_incr;
   case uint8('a')
      r(2)=q_incr;
   case uint8('d')
      r(2)=-q_incr;
   case uint8('q')
      r(3)=q_incr;
   case uint8('c')
      r(3)=-q_incr;
   otherwise
      x=zeros(1,3);
      r=zeros(1,3);
end

x_f=x;
r_f=r;

== matlab function External Object Forces/Apply Force/Embedded MATLAB Function1 ==
  data: xi input double size=[4 3]; RO output double
%#eml
function RO=R_O(xi)



x1 = xi(1,:);
x2 = xi(2,:);
x3 = xi(3,:);
x4 = xi(4,:);

% r1=( xi(1,:)-xi(3,:) )/norm( xi(1,:)-xi(3,:) ) + ...
%     ( xi(2,:)-xi(4,:) )/norm( xi(2,:)-xi(4,:) );

r1=( x1-x3 )/norm( x1-x3 ) + ...
    ( x2-x4 )/norm( x2-x4 );


r1_unit=r1/norm(r1);

% r3= cross( (x1-x3),( x2-x4 ))';

r3= skew( x1-x3 ) * ( x2-x4 )';
r3_unit=r3/norm(r3);

r2_unit = skew(r3_unit)*r1_unit';

l=[r1_unit' r2_unit r3_unit];
RO=l;

== matlab function External Object Forces/Apply Force/Embedded MATLAB Function2 ==
  data: q input double; x output double
%#eml
function x=x_i_v02(q)

x_=zeros(4,3);

rot_base=[0.0000         0   -1.0000;
         0    1.0000         0;
    1.0000         0    0.0000];

L1 = 0.10;
L2 = 1.10;
L3 = 0.60;
L4 = 0.55;

fingers_positions = [-0.70,   0,  L1;...
                      0.60,  0.40,  L1;...
                      0.70,   0,  L1;...
                      0.60,  -0.40, L1];

c=1;
                  
for i=1:4:16,

q1 = q(i);
q2 = q(i+1);
q3 = q(i+2);
q4 = q(i+3);

x_(c,1)=cos(q1) .* (L2 .* cos(q2) + L3 .* cos(q2 + q3) + L4 .*  cos(q2 + q3 + q4));
x_(c,2)=(L2 .* cos(q2) + L3 .* cos(q2 + q3) + L4 .* cos(q2 + q3 + q4)) .* sin(q1);
x_(c,3)= L2 .* sin(q2) + L3 .* sin(q2 + q3) + L4 .* sin(q2 + q3 + q4);

x_(c,:)=rot_base*x_(c,:)'+fingers_positions(c,:)';
c=c+1;
end

x=x_;

== matlab function External Object Forces/Apply Force/Embedded MATLAB Function ==
  data: u input double size=[4 3]; y output double
function y = fcn(u)
%#eml

y = ((u(1,:)+u(2,:)+u(3,:)+u(4,:))/4)';

== matlab function External Object Forces/Apply Torque/Subsystem/Embedded MATLAB Function ==
  data: u input double size=[4 3]; y output double
function y = fcn(u)
%#eml

y = ((u(1,:)+u(2,:)+u(3,:)+u(4,:))/4)';

== matlab function External Object Forces/Apply Torque/Subsystem/Embedded MATLAB Function1 ==
  data: xi input double size=[4 3]; RO output double
%#eml
function RO=R_O(xi)



x1 = xi(1,:);
x2 = xi(2,:);
x3 = xi(3,:);
x4 = xi(4,:);

% r1=( xi(1,:)-xi(3,:) )/norm( xi(1,:)-xi(3,:) ) + ...
%     ( xi(2,:)-xi(4,:) )/norm( xi(2,:)-xi(4,:) );

r1=( x1-x3 )/norm( x1-x3 ) + ...
    ( x2-x4 )/norm( x2-x4 );


r1_unit=r1/norm(r1);

% r3= cross( (x1-x3),( x2-x4 ))';

r3= skew( x1-x3 ) * ( x2-x4 )';
r3_unit=r3/norm(r3);

r2_unit = skew(r3_unit)*r1_unit';

l=[r1_unit' r2_unit r3_unit];
RO=l;

== matlab function External Object Forces/Apply Torque/Subsystem/Embedded MATLAB Function2 ==
  data: q input double; x output double
%#eml
function x=x_i_v02(q)

x_=zeros(4,3);

rot_base=[0.0000         0   -1.0000;
         0    1.0000         0;
    1.0000         0    0.0000];

L1 = 0.10;
L2 = 1.10;
L3 = 0.60;
L4 = 0.55;

fingers_positions = [-0.70,   0,  L1;...
                      0.60,  0.40,  L1;...
                      0.70,   0,  L1;...
                      0.60,  -0.40, L1];

c=1;
                  
for i=1:4:16,

q1 = q(i);
q2 = q(i+1);
q3 = q(i+2);
q4 = q(i+3);

x_(c,1)=cos(q1) .* (L2 .* cos(q2) + L3 .* cos(q2 + q3) + L4 .*  cos(q2 + q3 + q4));
x_(c,2)=(L2 .* cos(q2) + L3 .* cos(q2 + q3) + L4 .* cos(q2 + q3 + q4)) .* sin(q1);
x_(c,3)= L2 .* sin(q2) + L3 .* sin(q2 + q3) + L4 .* sin(q2 + q3 + q4);

x_(c,:)=rot_base*x_(c,:)'+fingers_positions(c,:)';
c=c+1;
end

x=x_;

== matlab function External Object Forces/Apply Torque/Subsystem2/Embedded MATLAB Function ==
  data: u input double size=[4 3]; y output double
function y = fcn(u)
%#eml

y = ((u(1,:)+u(2,:)+u(3,:)+u(4,:))/4)';

== matlab function External Object Forces/Apply Torque/Subsystem2/Embedded MATLAB Function1 ==
  data: xi input double size=[4 3]; RO output double
%#eml
function RO=R_O(xi)



x1 = xi(1,:);
x2 = xi(2,:);
x3 = xi(3,:);
x4 = xi(4,:);

% r1=( xi(1,:)-xi(3,:) )/norm( xi(1,:)-xi(3,:) ) + ...
%     ( xi(2,:)-xi(4,:) )/norm( xi(2,:)-xi(4,:) );

r1=( x1-x3 )/norm( x1-x3 ) + ...
    ( x2-x4 )/norm( x2-x4 );


r1_unit=r1/norm(r1);

% r3= cross( (x1-x3),( x2-x4 ))';

r3= skew( x1-x3 ) * ( x2-x4 )';
r3_unit=r3/norm(r3);

r2_unit = skew(r3_unit)*r1_unit';

l=[r1_unit' r2_unit r3_unit];
RO=l;

== matlab function External Object Forces/Apply Torque/Subsystem2/Embedded MATLAB Function2 ==
  data: q input double; x output double
%#eml
function x=x_i_v02(q)

x_=zeros(4,3);

rot_base=[0.0000         0   -1.0000;
         0    1.0000         0;
    1.0000         0    0.0000];

L1 = 0.10;
L2 = 1.10;
L3 = 0.60;
L4 = 0.55;

fingers_positions = [-0.70,   0,  L1;...
                      0.60,  0.40,  L1;...
                      0.70,   0,  L1;...
                      0.60,  -0.40, L1];

c=1;
                  
for i=1:4:16,

q1 = q(i);
q2 = q(i+1);
q3 = q(i+2);
q4 = q(i+3);

x_(c,1)=cos(q1) .* (L2 .* cos(q2) + L3 .* cos(q2 + q3) + L4 .*  cos(q2 + q3 + q4));
x_(c,2)=(L2 .* cos(q2) + L3 .* cos(q2 + q3) + L4 .* cos(q2 + q3 + q4)) .* sin(q1);
x_(c,3)= L2 .* sin(q2) + L3 .* sin(q2 + q3) + L4 .* sin(q2 + q3 + q4);

x_(c,:)=rot_base*x_(c,:)'+fingers_positions(c,:)';
c=c+1;
end

x=x_;

== matlab function Control/IPC/Embedded MATLAB Function ==
  data: theta_in input double; gravity_dynamic_term output double
function gravity_dynamic_term = gravity_dynamic_term(theta_in)

c= zeros(1,16);
g= 9.81;

gain=1.1;

DOFs = 16;

L1 = 0.10;
L2 = 1.10;
L3 = 0.60;
L4 = 0.55;


caspule1mass = 2.00;
caspule2mass = 1.00;
caspule3mass = 1.00;


for i=1:4:DOFs,
q1=theta_in(i);
q2=theta_in(i+1);
q3=theta_in(i+2);
q4=theta_in(i+3);

c(i:i+3)=gain*[(-1 / 2) .* g .* ((caspule1mass .* L2 + 2 .* caspule2mass .* L2 + ...
   2 .* caspule3mass .* L2) .* cos(q2) + (caspule2mass .* L3 + 2 .*  ...
  caspule3mass .* L3) .* cos(q2 + q3) + caspule3mass .* L4 .* cos( ...
  q2 + q3 + q4)) .* sin(q1),(-1 / 2) .* g .* cos(q1) .* (( ...
  caspule1mass .* L2 + 2 .* caspule2mass .* L2 + 2 .* caspule3mass  ...
  .* L2) .* sin(q2) + (caspule2mass .* L3 + 2 .* caspule3mass .* L3) ...
   .* sin(q2 + q3) + caspule3mass .* L4 .* sin(q2 + q3 + q4)),(-1 /  ...
  2) .* g .* cos(q1) .* ((caspule2mass .* L3 + 2 .* caspule3mass .*  ...
  L3) .* sin(q2 + q3) + caspule3mass .* L4 .* sin(q2 + q3 + q4)),( ...
  -1 / 2) .* caspule3mass .* g .* L4 .* cos(q1) .* sin(q2 + q3 + q4) ...
  ];
end

gravity_dynamic_term=c;
